simulink model "sistema_fisico_test"  (R2019a)
settings: Solver=VariableStepAuto  StartTime=0.0  StopTime=240  RelTol=1e-3
undefined symbols (not defined in the file): b_cx, b_cy, b_h_eq, b_hb, b_hEb, b_t, b_tb, b_td_eq, b_tw, b_wu, g, H_c, i_h, i_t, K_cy, K_tw, k_wu, l_h0, m_h_eq, M_t, m_td_eq, r_hd, r_td, sigbuilder_block, T_hb_max, T_hEb_max, T_tb_max, x_l0, x_t0, x_td0, y_l0, Y_t0
libraries: simulink x1
settings Model: Creator=Facundo  LastModifiedBy=Facundo

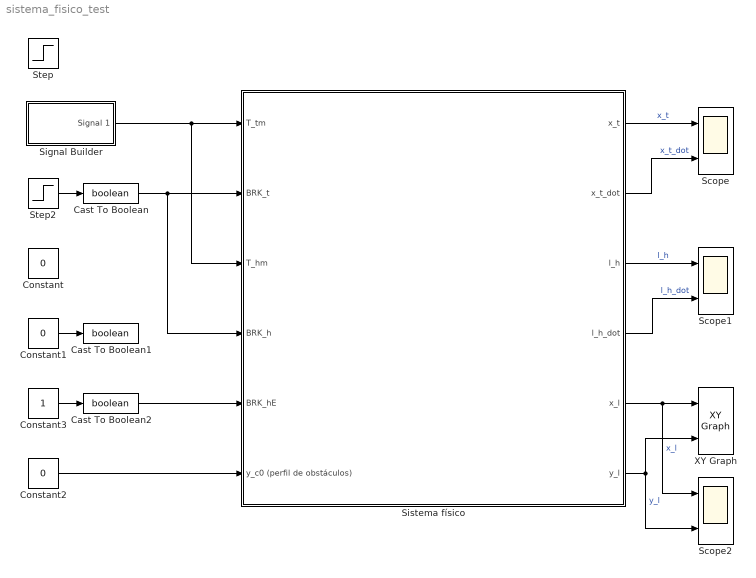
== system sistema_fisico_test ==
  Cast To Boolean : DataTypeConversion  OutDataTypeStr=boolean
  Cast To Boolean1 : DataTypeConversion  OutDataTypeStr=boolean
  Cast To Boolean2 : DataTypeConversion  OutDataTypeStr=boolean
  Constant : Constant  Value=0
  Constant1 : Constant  Value=0  OutDataTypeStr=boolean
  Constant2 : Constant  Value=0
  Constant3 : Constant  OutDataTypeStr=boolean
  Scope : Scope  NumInputPorts=2
  Scope1 : Scope  NumInputPorts=2
  Scope2 : Scope  NumInputPorts=2
  Signal Builder : Subsystem  Tag=STV Subsys  LoadFcn=sigbuilder_block('load');  StartFcn=sigbuilder_block('start');  StopFcn=sigbuilder_block('stop');  ClipboardFcn=sigbuilder_block('clipboard');  mask(Sigbuilder block){tuvar=[0:10]}
      mask help: Simulink:masks:SigbuilderBlock_MD
      mask init:
      | if ~strcmp(get_param(bdroot(gcbh),'SimulationStatus'),'stopped') tuvar = sigbuilder_block('maskInit'); end
      settings: CopyFcn=sigbuilder_block('copy');  DeleteFcn=sigbuilder_block('delete');  ModelCloseFcn=sigbuilder_block('modelClose');  PreSaveFcn=sigbuilder_block('preSave');  PauseFcn=sigbuilder_block('pause');  ContinueFcn=sigbuilder_block('continue');  NameChangeFcn=sigbuilder_block('namechange');  OpenFcn=sigbuilder_block('open',[-1440 -265.714 1440 726.429 ]);  CloseFcn=sigbuilder_block('close');
      mask Display: plot(0, 0, 100, 100,[2, 2, 32, 32, 2], [68, 8, 8, 68, 68],[32, 2], [38, 38], [32, 19, 2],[53, 60, 44], [32, 17, 17, 2],[16, 16, 31, 31]);txt = getActiveGroup(gcbh);text(2, 100, txt,'verticalAlignment', 'top');
  Sistema físico : Subsystem
  Step : Step  Time=0.5  After=1000  SampleTime=0
  Step2 : Step  Time=25  Before=1  After=0  SampleTime=0
  XY Graph : simulink/Sinks/XY Graph  xmin=-100  xmax=100  ymin=-100  ymax=100  st=-1
  wires:
  Constant2/1 -> Sistema físico/6(y_c0 (perfil de obstáculos))
  Constant1/1 -> Cast To Boolean1/1
  Step2/1 -> Cast To Boolean/1
  Sistema físico/2(x_t_dot) -> Scope/2  "x_t_dot"
  Sistema físico/3(l_h) -> Scope1/1  "l_h"
  Sistema físico/5(x_l) -> XY Graph/1, Scope2/1  "x_l"
  Sistema físico/6(y_l) -> Scope2/2, XY Graph/2  "y_l"
  Sistema físico/4(l_h_dot) -> Scope1/2  "l_h_dot"
  Sistema físico/1(x_t) -> Scope/1  "x_t"
  Signal Builder/1(Signal 1) -> Sistema físico/1(T_tm), Sistema físico/3(T_hm)
  Constant3/1 -> Cast To Boolean2/1
  Cast To Boolean2/1 -> Sistema físico/5(BRK_hE)
  Cast To Boolean/1 -> Sistema físico/4(BRK_h), Sistema físico/2(BRK_t)

== system sistema_fisico_test/Signal Builder ==
  Demux : Demux  Tag=STV Demux  Outputs=1
  FromWs : FromWorkspace  Tag=STV FromWs  VariableName=tuvar  SampleTime=0
      SigBuilderData=|
      | common.afterFinalStr = 'Extrapolate'
      | common.sampleTime = 0
      | dataSet.timeRange = [0 60]
      | dataSet.name = 'Group 1'
      | sbobj.Groups.Name = 'Group 1'
      | sbobj.Groups.Signals.Name = 'Signal 1'
      | sbobj.Groups.Signals.XData = [0 1 10 30 60]
      | sbobj.Groups.Signals.YData = [0 1000 1000 0 0]
      | sbobj.Groups.TimeRange = [0 60]
  Signal 1 : Outport  Tag=STV Outport
  wires:
  Demux/1 -> Signal 1/1
  FromWs/1 -> Demux/1

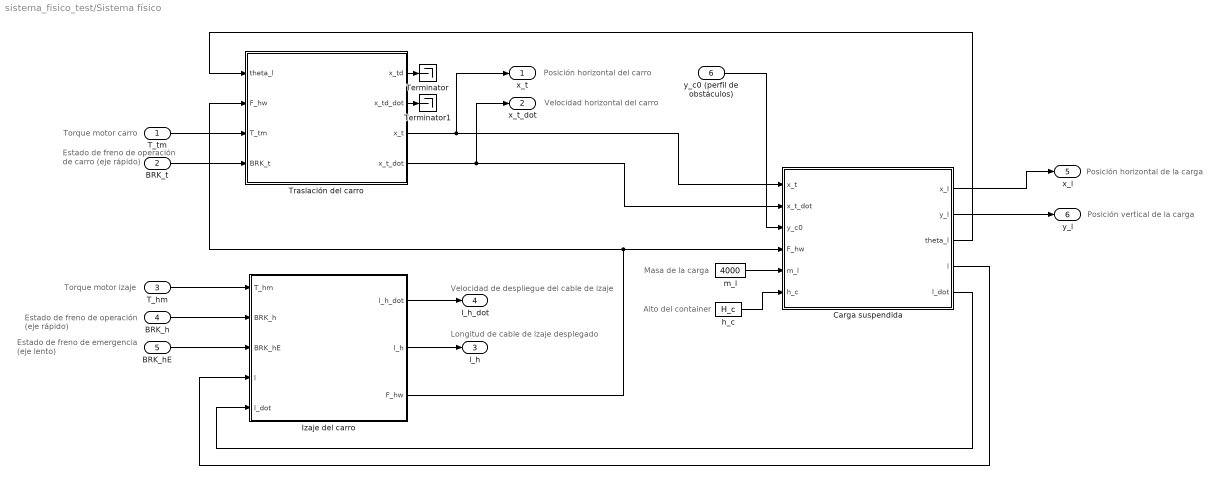
== system sistema_fisico_test/Sistema físico ==
  note: Alto del container
  note: Masa de la carga
  note: Torque motor izaje
  note: Estado de freno de operación
      | (eje rápido)
  note: Estado de freno de emergencia
      | (eje lento)
  note: Estado de freno de
      | operación de carro
      | (eje rápido)
  note: Torque motor carro
  note: Posición vertical de la carga
  note: Posición horizontal de la carga
  note: Longitud de cable de izaje desplegado
  note: Velocidad de despliegue del cable de izaje
  note: Posición horizontal del carro
  note: Velocidad horizontal del carro
  T_tm : Inport
  BRK_t : Inport  Port=2
  T_hm : Inport  Port=3
  BRK_h : Inport  Port=4
  BRK_hE : Inport  Port=5
  y_c0 (perfil de obstáculos) : Inport  Port=6
  Carga suspendida : Subsystem
  Izaje del carro : Subsystem
  Terminator : Terminator
  Terminator1 : Terminator
  Traslación del carro : Subsystem
  h_c : Constant  Value=H_c
  m_l : Constant  Value=4000
  x_t : Outport
  x_t_dot : Outport  Port=2
  l_h : Outport  Port=3
  l_h_dot : Outport  Port=4
  x_l : Outport  Port=5
  y_l : Outport  Port=6
  wires:
  Carga suspendida/5(l_dot) -> Izaje del carro/5(l_dot)
  Traslación del carro/3(x_t) -> x_t/1, Carga suspendida/1(x_t)
  Carga suspendida/2(y_l) -> y_l/1
  Traslación del carro/2(x_td_dot) -> Terminator1/1
  BRK_h/1 -> Izaje del carro/2(BRK_h)
  Izaje del carro/2(l_h) -> l_h/1
  Izaje del carro/1(l_h_dot) -> l_h_dot/1
  m_l/1 -> Carga suspendida/5(m_l)
  Carga suspendida/4(l) -> Izaje del carro/4(l)
  Carga suspendida/1(x_l) -> x_l/1
  Izaje del carro/3(F_hw) -> Traslación del carro/2(F_hw), Carga suspendida/4(F_hw)
  Traslación del carro/4(x_t_dot) -> x_t_dot/1, Carga suspendida/2(x_t_dot)
  BRK_t/1 -> Traslación del carro/4(BRK_t)
  h_c/1 -> Carga suspendida/6(h_c)
  y_c0 (perfil de obstáculos)/1 -> Carga suspendida/3(y_c0)
  BRK_hE/1 -> Izaje del carro/3(BRK_hE)
  Traslación del carro/1(x_td) -> Terminator/1
  T_hm/1 -> Izaje del carro/1(T_hm)
  T_tm/1 -> Traslación del carro/3(T_tm)
  Carga suspendida/3(theta_l) -> Traslación del carro/1(theta_l)

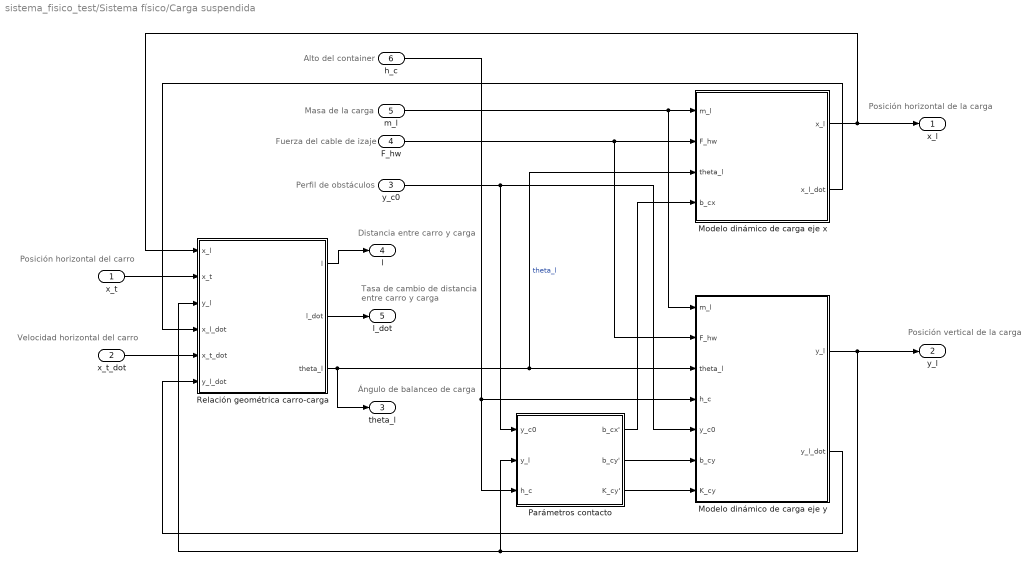
== system sistema_fisico_test/Sistema físico/Carga suspendida ==
  note: Perfil de obstáculos
  note: Posición horizontal del carro
  note: Posición vertical de la carga
  note: Velocidad horizontal del carro
  note: Alto del container
  note: Distancia entre carro y carga
  note: Fuerza del cable de izaje
  note: Ángulo de balanceo de carga
  note: Tasa de cambio de distancia
      | entre carro y carga
  note: Masa de la carga
  note: Posición horizontal de la carga
  x_t : Inport  OutDataTypeStr=double  PortDimensions=1  SampleTime=0
  x_t_dot : Inport  Port=2  OutDataTypeStr=double  PortDimensions=1  SampleTime=0
  y_c0 : Inport  Port=3  OutDataTypeStr=double  PortDimensions=1  SampleTime=0
  F_hw : Inport  Port=4  OutDataTypeStr=double  PortDimensions=1  SampleTime=0
  m_l : Inport  Port=5  OutDataTypeStr=double  PortDimensions=1  SampleTime=0
  h_c : Inport  Port=6  OutDataTypeStr=double  PortDimensions=1  SampleTime=0
  Modelo dinámico de carga eje x : Subsystem
  Modelo dinámico de carga eje y : Subsystem
  Parámetros contacto : Subsystem
  Relación geométrica carro-carga : Subsystem
  x_l : Outport  OutDataTypeStr=double  PortDimensions=1  SampleTime=0
  y_l : Outport  Port=2  OutDataTypeStr=double  PortDimensions=1  SampleTime=0
  theta_l : Outport  Port=3  OutDataTypeStr=double  PortDimensions=1  SampleTime=0
  l : Outport  Port=4  OutDataTypeStr=double  PortDimensions=1  SampleTime=0
  l_dot : Outport  Port=5  OutDataTypeStr=double  PortDimensions=1  SampleTime=0
  wires:
  y_c0/1 -> Parámetros contacto/1(y_c0), Modelo dinámico de carga eje y/5(y_c0)
  m_l/1 -> Modelo dinámico de carga eje y/1(m_l), Modelo dinámico de carga eje x/1(m_l)
  F_hw/1 -> Modelo dinámico de carga eje y/2(F_hw), Modelo dinámico de carga eje x/2(F_hw)
  Relación geométrica carro-carga/2(l_dot) -> l_dot/1
  x_t_dot/1 -> Relación geométrica carro-carga/5(x_t_dot)
  Modelo dinámico de carga eje y/1(y_l) -> y_l/1, Relación geométrica carro-carga/3(y_l), Parámetros contacto/2(y_l)
  h_c/1 -> Modelo dinámico de carga eje y/4(h_c), Parámetros contacto/3(h_c)
  Modelo dinámico de carga eje x/2(x_l_dot) -> Relación geométrica carro-carga/4(x_l_dot)
  Modelo dinámico de carga eje y/2(y_l_dot) -> Relación geométrica carro-carga/6(y_l_dot)
  x_t/1 -> Relación geométrica carro-carga/2(x_t)
  Modelo dinámico de carga eje x/1(x_l) -> x_l/1, Relación geométrica carro-carga/1(x_l)
  Relación geométrica carro-carga/3(theta_l) -> theta_l/1, Modelo dinámico de carga eje x/3(theta_l), Modelo dinámico de carga eje y/3(theta_l)  "theta_l"
  Parámetros contacto/1(b_cx') -> Modelo dinámico de carga eje x/4(b_cx)
  Parámetros contacto/2(b_cy') -> Modelo dinámico de carga eje y/6(b_cy)
  Parámetros contacto/3(K_cy') -> Modelo dinámico de carga eje y/7(K_cy)
  Relación geométrica carro-carga/1(l) -> l/1

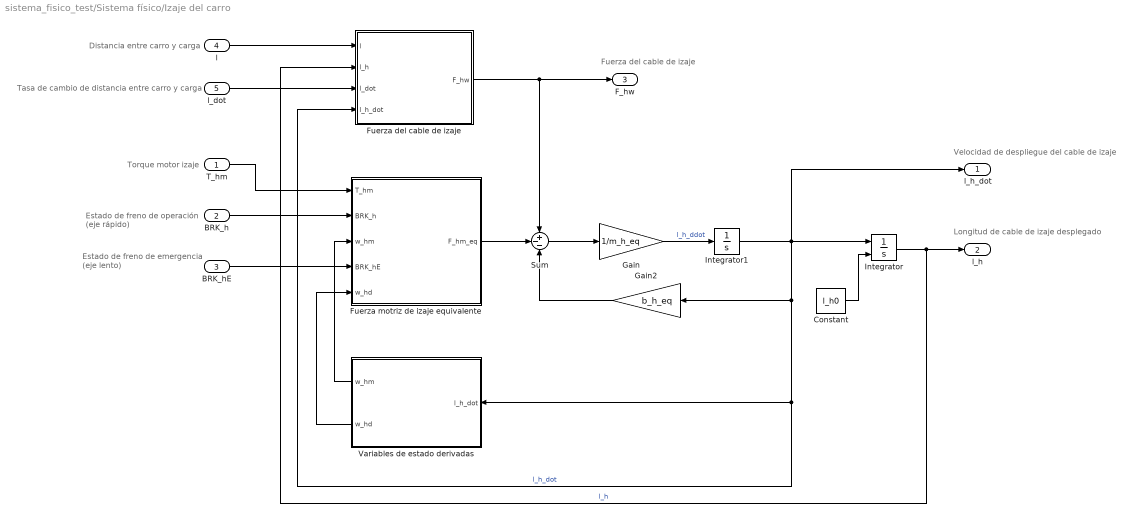
== system sistema_fisico_test/Sistema físico/Izaje del carro ==
  note: Longitud de cable de izaje desplegado
  note: Velocidad de despliegue del cable de izaje
  note: Torque motor izaje
  note: Estado de freno de emergencia
      | (eje lento)
  note: Tasa de cambio de distancia entre carro y carga
  note: Estado de freno de operación
      | (eje rápido)
  note: Distancia entre carro y carga
  note: Fuerza del cable de izaje
  T_hm : Inport
  BRK_h : Inport  Port=2
  BRK_hE : Inport  Port=3
  l : Inport  Port=4
  l_dot : Inport  Port=5
  Constant : Constant  Value=l_h0
  Fuerza del cable de izaje : Subsystem
  Fuerza motriz de izaje equivalente : Subsystem
  Gain : Gain  Gain=1/m_h_eq
  Gain2 : Gain  Gain=b_h_eq
  Integrator : Integrator  InitialConditionSource=external
  Integrator1 : Integrator
  Sum : Sum  Inputs=+--
  Variables de estado derivadas : Subsystem
  l_h_dot : Outport
  l_h : Outport  Port=2
  F_hw : Outport  Port=3
  wires:
  Integrator/1 -> l_h/1, Fuerza del cable de izaje/2(l_h)  "l_h"
  Integrator1/1 -> l_h_dot/1, Fuerza del cable de izaje/4(l_h_dot), Variables de estado derivadas/1(l_h_dot), Gain2/1, Integrator/1  "l_h_dot"
  T_hm/1 -> Fuerza motriz de izaje equivalente/1(T_hm)
  l/1 -> Fuerza del cable de izaje/1(l)
  l_dot/1 -> Fuerza del cable de izaje/3(l_dot)
  Fuerza del cable de izaje/1(F_hw) -> F_hw/1, Sum/1
  Gain2/1 -> Sum/3
  Fuerza motriz de izaje equivalente/1(F_hm_eq) -> Sum/2
  Variables de estado derivadas/1(w_hm) -> Fuerza motriz de izaje equivalente/3(w_hm)
  Sum/1 -> Gain/1
  Variables de estado derivadas/2(w_hd) -> Fuerza motriz de izaje equivalente/5(w_hd)
  BRK_h/1 -> Fuerza motriz de izaje equivalente/2(BRK_h)
  BRK_hE/1 -> Fuerza motriz de izaje equivalente/4(BRK_hE)
  Gain/1 -> Integrator1/1  "l_h_ddot"
  Constant/1 -> Integrator/2

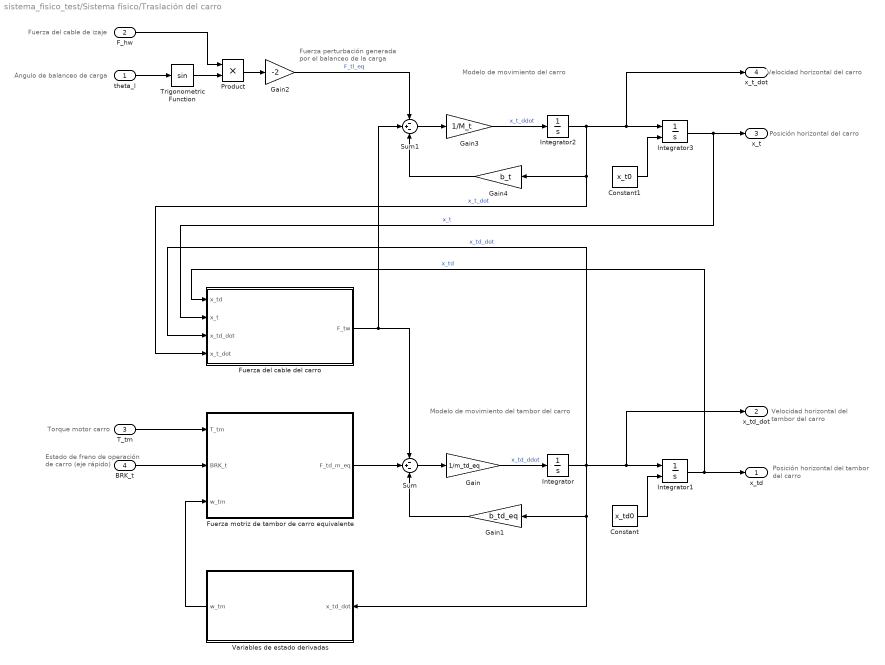
== system sistema_fisico_test/Sistema físico/Traslación del carro ==
  note: Velocidad horizontal
      | del tambor del carro
  note: Modelo de movimiento del tambor del carro
  note: Modelo de movimiento del carro
  note: Velocidad horizontal del carro
  note: Estado de freno de
      | operación de carro
      | (eje rápido)
  note: Fuerza del cable de izaje
  note: Fuerza perturbación generada
      | por el balanceo de la carga
  note: Posición horizontal del carro
  note: Torque motor carro
  note: Ángulo de balanceo de carga
  note: Posición horizontal
      | del tambor del carro
  theta_l : Inport  OutDataTypeStr=double  PortDimensions=1  SampleTime=0
  F_hw : Inport  Port=2  OutDataTypeStr=double  PortDimensions=1  SampleTime=0
  T_tm : Inport  Port=3
  BRK_t : Inport  Port=4
  Constant : Constant  Value=x_td0
  Constant1 : Constant  Value=x_t0
  Fuerza del cable del carro : Subsystem
  Fuerza motriz de tambor de carro equivalente : Subsystem
  Gain : Gain  Gain=1/m_td_eq
  Gain1 : Gain  Gain=b_td_eq
  Gain2 : Gain  Gain=-2
  Gain3 : Gain  Gain=1/M_t
  Gain4 : Gain  Gain=b_t
  Integrator : Integrator
  Integrator1 : Integrator  InitialConditionSource=external
  Integrator2 : Integrator
  Integrator3 : Integrator  InitialConditionSource=external
  Product : Product
  Sum : Sum  Inputs=-+-
  Sum1 : Sum  Inputs=-+-
  Trigonometric Function : Trigonometry
  Variables de estado derivadas : Subsystem
  x_td : Outport  OutDataTypeStr=double  PortDimensions=1  SampleTime=0
  x_td_dot : Outport  Port=2  OutDataTypeStr=double  PortDimensions=1  SampleTime=0
  x_t : Outport  Port=3  OutDataTypeStr=double  PortDimensions=1  SampleTime=0
  x_t_dot : Outport  Port=4  OutDataTypeStr=double  PortDimensions=1  SampleTime=0
  wires:
  Integrator1/1 -> x_td/1, Fuerza del cable del carro/1(x_td)  "x_td"
  Gain3/1 -> Integrator2/1  "x_t_ddot"
  Fuerza del cable del carro/1(F_tw) -> Sum1/2, Sum/1
  Sum/1 -> Gain/1
  Integrator/1 -> Fuerza del cable del carro/3(x_td_dot), Variables de estado derivadas/1(x_td_dot), Gain1/1, x_td_dot/1, Integrator1/1  "x_td_dot"
  F_hw/1 -> Product/1
  Fuerza motriz de tambor de carro equivalente/1(F_td_m_eq) -> Sum/2
  Constant/1 -> Integrator1/2
  Gain1/1 -> Sum/3
  Integrator2/1 -> Fuerza del cable del carro/4(x_t_dot), Gain4/1, x_t_dot/1, Integrator3/1  "x_t_dot"
  Sum1/1 -> Gain3/1
  theta_l/1 -> Trigonometric Function/1
  Gain4/1 -> Sum1/3
  Integrator3/1 -> x_t/1, Fuerza del cable del carro/2(x_t)  "x_t"
  Gain2/1 -> Sum1/1  "F_tl_eq"
  T_tm/1 -> Fuerza motriz de tambor de carro equivalente/1(T_tm)
  BRK_t/1 -> Fuerza motriz de tambor de carro equivalente/2(BRK_t)
  Variables de estado derivadas/1(w_tm) -> Fuerza motriz de tambor de carro equivalente/3(w_tm)
  Constant1/1 -> Integrator3/2
  Trigonometric Function/1 -> Product/2
  Product/1 -> Gain2/1
  Gain/1 -> Integrator/1  "x_td_ddot"

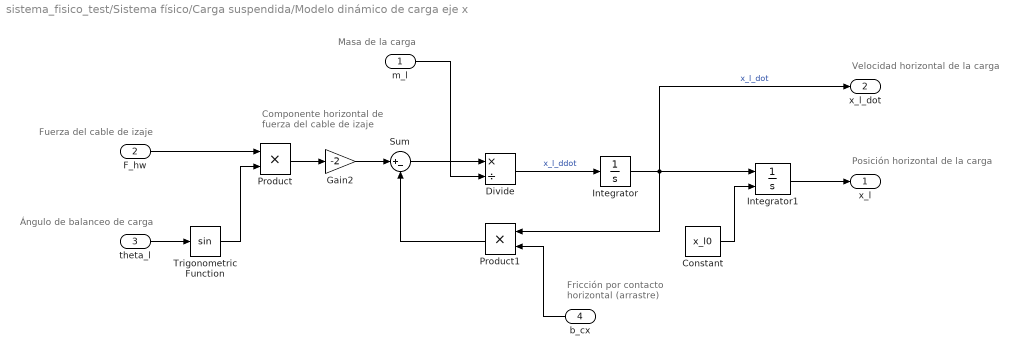
== system sistema_fisico_test/Sistema físico/Carga suspendida/Modelo dinámico de carga eje x ==
  note: Componente horizontal de
      | fuerza del cable de izaje
  note: Posición horizontal de la carga
  note: Velocidad horizontal de la carga
  note: Fuerza del cable de izaje
  note: Masa de la carga
  note: Fricción por contacto
      | horizontal (arrastre)
  note: Ángulo de balanceo de carga
  m_l : Inport  OutDataTypeStr=double  PortDimensions=1  SampleTime=0
  F_hw : Inport  Port=2  OutDataTypeStr=double  PortDimensions=1  SampleTime=0
  theta_l : Inport  Port=3  OutDataTypeStr=double  PortDimensions=1  SampleTime=0
  b_cx : Inport  Port=4  OutDataTypeStr=double  PortDimensions=1  SampleTime=0
  Constant : Constant  Value=x_l0
  Divide : Product  Inputs=*/
  Gain2 : Gain  Gain=-2
  Integrator : Integrator
  Integrator1 : Integrator  InitialConditionSource=external
  Product : Product
  Product1 : Product
  Sum : Sum  Inputs=|+-
  Trigonometric Function : Trigonometry
  x_l : Outport  OutDataTypeStr=double  PortDimensions=1  SampleTime=0
  x_l_dot : Outport  Port=2  OutDataTypeStr=double  PortDimensions=1  SampleTime=0
  wires:
  F_hw/1 -> Product/1
  Product1/1 -> Sum/2
  theta_l/1 -> Trigonometric Function/1
  b_cx/1 -> Product1/2
  Sum/1 -> Divide/1
  Integrator/1 -> x_l_dot/1, Integrator1/1, Product1/1  "x_l_dot"
  Product/1 -> Gain2/1
  Divide/1 -> Integrator/1  "x_l_ddot"
  Constant/1 -> Integrator1/2
  Integrator1/1 -> x_l/1
  Gain2/1 -> Sum/1
  m_l/1 -> Divide/2
  Trigonometric Function/1 -> Product/2

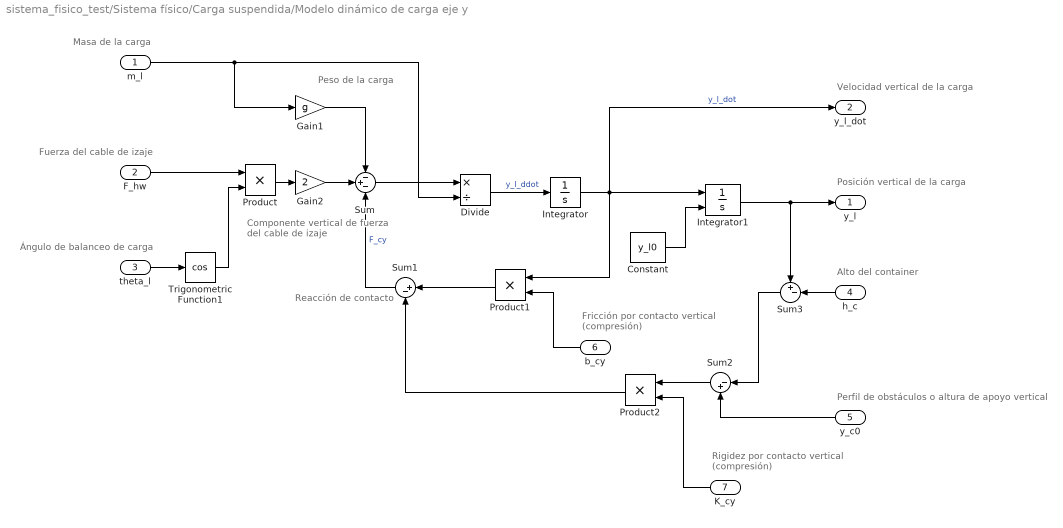
== system sistema_fisico_test/Sistema físico/Carga suspendida/Modelo dinámico de carga eje y ==
  note: Reacción de contacto
  note: Peso de la carga
  note: Componente vertical de
      | fuerza del cable de izaje
  note: Posición vertical de la carga
  note: Velocidad vertical de la carga
  note: Fricción por contacto
      | vertical (compresión)
  note: Rigidez por contacto
      | vertical (compresión)
  note: Masa de la carga
  note: Fuerza del cable de izaje
  note: Perfil de obstáculos o altura de apoyo vertical
  note: Alto del container
  note: Ángulo de balanceo de carga
  m_l : Inport  OutDataTypeStr=double  PortDimensions=1  SampleTime=0
  F_hw : Inport  Port=2  OutDataTypeStr=double  PortDimensions=1  SampleTime=0
  theta_l : Inport  Port=3  OutDataTypeStr=double  PortDimensions=1  SampleTime=0
  h_c : Inport  Port=4  OutDataTypeStr=double  PortDimensions=1  SampleTime=0
  y_c0 : Inport  Port=5  OutDataTypeStr=double  PortDimensions=1  SampleTime=0
  b_cy : Inport  Port=6  OutDataTypeStr=double  PortDimensions=1  SampleTime=0
  K_cy : Inport  Port=7  OutDataTypeStr=double  PortDimensions=1  SampleTime=0
  Constant : Constant  Value=y_l0
  Divide : Product  Inputs=*/
  Gain1 : Gain  Gain=g
  Gain2 : Gain  Gain=2
  Integrator : Integrator
  Integrator1 : Integrator  InitialConditionSource=external
  Product : Product
  Product1 : Product
  Product2 : Product
  Sum : Sum  Inputs=-+-
  Sum1 : Sum  Inputs=|+-
  Sum2 : Sum  Inputs=|-+
  Sum3 : Sum  Inputs=+-|
  Trigonometric Function1 : Trigonometry  Operator=cos
  y_l : Outport  OutDataTypeStr=double  PortDimensions=1  SampleTime=0
  y_l_dot : Outport  Port=2  OutDataTypeStr=double  PortDimensions=1  SampleTime=0
  wires:
  F_hw/1 -> Product/1
  theta_l/1 -> Trigonometric Function1/1
  b_cy/1 -> Product1/2
  Integrator/1 -> y_l_dot/1, Integrator1/1, Product1/1  "y_l_dot"
  Divide/1 -> Integrator/1  "y_l_ddot"
  Constant/1 -> Integrator1/2
  Integrator1/1 -> y_l/1, Sum3/1
  Product/1 -> Gain2/1
  Product1/1 -> Sum1/1
  Sum1/1 -> Sum/3  "F_cy"
  Gain1/1 -> Sum/1
  y_c0/1 -> Sum2/2
  Sum2/1 -> Product2/1
  K_cy/1 -> Product2/2
  Product2/1 -> Sum1/2
  Gain2/1 -> Sum/2
  Sum/1 -> Divide/1
  m_l/1 -> Gain1/1, Divide/2
  h_c/1 -> Sum3/2
  Sum3/1 -> Sum2/1
  Trigonometric Function1/1 -> Product/2

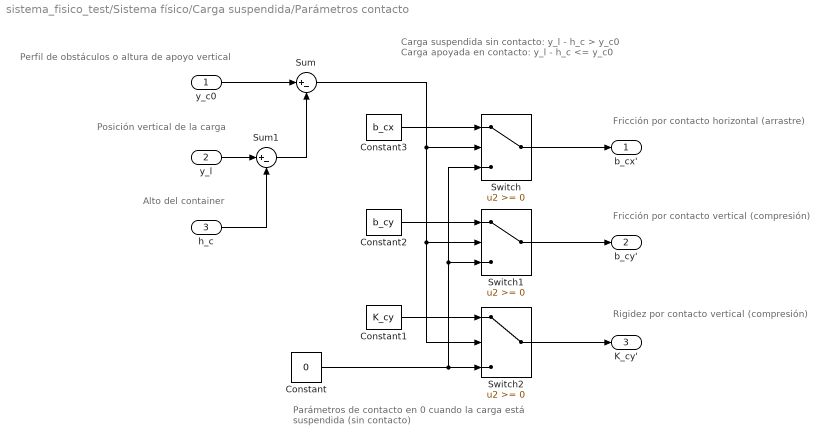
== system sistema_fisico_test/Sistema físico/Carga suspendida/Parámetros contacto ==
  note: Fricción por contacto horizontal (arrastre)
  note: Fricción por contacto vertical (compresión)
  note: Rigidez por contacto vertical (compresión)
  note: Perfil de obstáculos o altura de apoyo vertical
  note: Posición vertical de la carga
  note: Alto del container
  note: Parámetros de contacto en 0
      | cuando la carga está suspendida (sin contacto)
  note: Carga suspendida sin contacto: y_l - h_c > y_c0
      | Carga apoyada en contacto: y_l - h_c <= y_c0
  y_c0 : Inport  OutDataTypeStr=double  PortDimensions=1  SampleTime=0
  y_l : Inport  Port=2  OutDataTypeStr=double  PortDimensions=1  SampleTime=0
  h_c : Inport  Port=3  OutDataTypeStr=double  PortDimensions=1  SampleTime=0
  Constant : Constant  Value=0
  Constant1 : Constant  Value=K_cy
  Constant2 : Constant  Value=b_cy
  Constant3 : Constant  Value=b_cx
  Sum : Sum  Inputs=|+-
  Sum1 : Sum  Inputs=|+-
  Switch : Switch
  Switch1 : Switch
  Switch2 : Switch
  b_cx' : Outport  OutDataTypeStr=double  PortDimensions=1  SampleTime=0
  b_cy' : Outport  Port=2  OutDataTypeStr=double  PortDimensions=1  SampleTime=0
  K_cy' : Outport  Port=3  OutDataTypeStr=double  PortDimensions=1  SampleTime=0
  wires:
  y_c0/1 -> Sum/1
  Constant2/1 -> Switch1/1
  Constant1/1 -> Switch2/1
  Switch/1 -> b_cx'/1
  Sum/1 -> Switch1/2, Switch2/2, Switch/2
  Switch2/1 -> K_cy'/1
  Switch1/1 -> b_cy'/1
  Constant/1 -> Switch/3, Switch1/3, Switch2/3
  Constant3/1 -> Switch/1
  Sum1/1 -> Sum/2
  y_l/1 -> Sum1/1
  h_c/1 -> Sum1/2

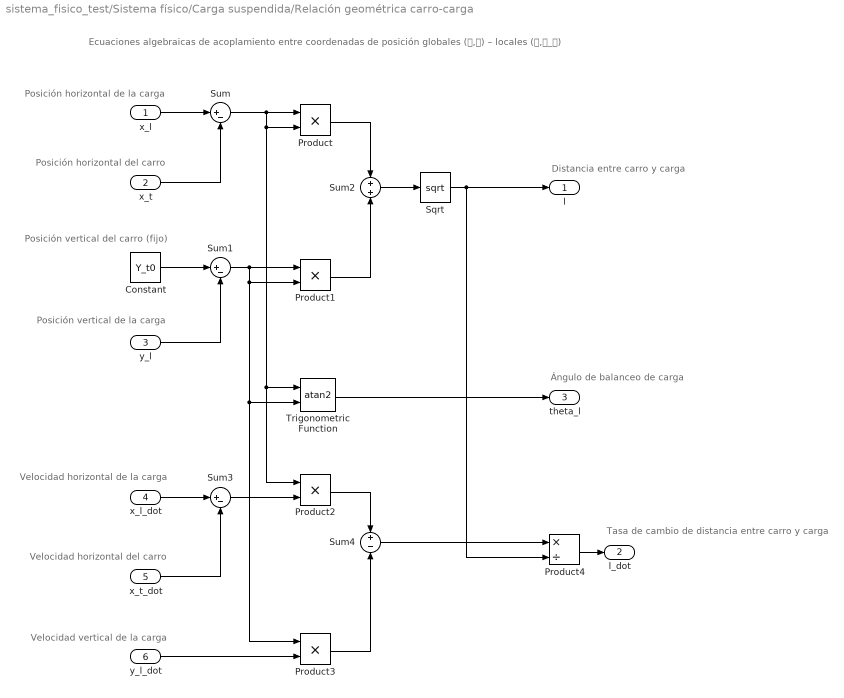
== system sistema_fisico_test/Sistema físico/Carga suspendida/Relación geométrica carro-carga ==
  note: Ecuaciones algebraicas de acoplamiento entre coordenadas de posición globales (𝑥,𝑦) – locales (𝑙,𝜃_𝑙)
  note: Posición horizontal de la carga
  note: Posición horizontal del carro
  note: Posición vertical del carro (fijo)
  note: Posición vertical de la carga
  note: Distancia entre carro y carga
  note: Tasa de cambio de distancia entre carro y carga
  note: Ángulo de balanceo de carga
  note: Velocidad horizontal de la carga
  note: Velocidad horizontal del carro
  note: Velocidad vertical de la carga
  x_l : Inport
  x_t : Inport  Port=2
  y_l : Inport  Port=3
  x_l_dot : Inport  Port=4
  x_t_dot : Inport  Port=5
  y_l_dot : Inport  Port=6
  Constant : Constant  Value=Y_t0
  Product{,1..3} (4 alike) : Product
  Product4 : Product  Inputs=*/
  Sqrt : Sqrt  SaturateOnIntegerOverflow=on
  Sum : Sum  Inputs=|+-
  Sum1 : Sum  Inputs=|+-
  Sum2 : Sum  Inputs=+|+
  Sum3 : Sum  Inputs=|+-
  Sum4 : Sum  Inputs=+|-
  Trigonometric Function : Trigonometry  Operator=atan2
  l : Outport
  l_dot : Outport  Port=2
  theta_l : Outport  Port=3
  wires:
  x_t/1 -> Sum/2
  x_l/1 -> Sum/1
  Sum/1 -> Product/1, Product2/1, Trigonometric Function/1, Product/2
  Product/1 -> Sum2/1
  y_l/1 -> Sum1/2
  Sum1/1 -> Product1/1, Product3/1, Trigonometric Function/2, Product1/2
  Constant/1 -> Sum1/1
  Product1/1 -> Sum2/2
  Sum2/1 -> Sqrt/1
  Trigonometric Function/1 -> theta_l/1
  x_l_dot/1 -> Sum3/1
  x_t_dot/1 -> Sum3/2
  Sum3/1 -> Product2/2
  y_l_dot/1 -> Product3/2
  Product2/1 -> Sum4/1
  Product3/1 -> Sum4/2
  Sum4/1 -> Product4/1
  Product4/1 -> l_dot/1
  Sqrt/1 -> Product4/2, l/1

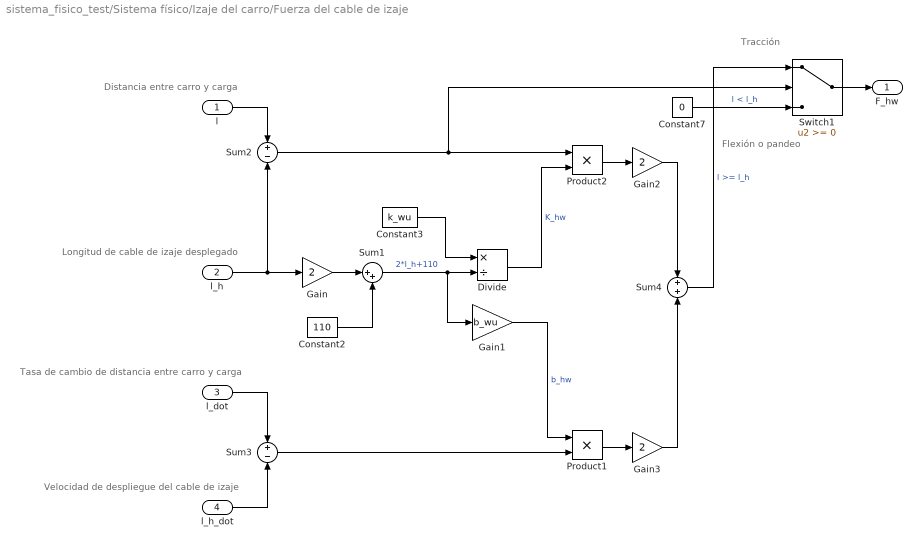
== system sistema_fisico_test/Sistema físico/Izaje del carro/Fuerza del cable de izaje ==
  note: Flexión o pandeo
  note: Tracción
  note: Distancia entre carro y carga
  note: Tasa de cambio de distancia entre carro y carga
  note: Longitud de cable de izaje desplegado
  note: Velocidad de despliegue del cable de izaje
  l : Inport
  l_h : Inport  Port=2
  l_dot : Inport  Port=3
  l_h_dot : Inport  Port=4
  Constant2 : Constant  Value=110
  Constant3 : Constant  Value=k_wu
  Constant7 : Constant  Value=0
  Divide : Product  Inputs=*/
  Gain : Gain  Gain=2
  Gain1 : Gain  Gain=b_wu
  Gain2 : Gain  Gain=2
  Gain3 : Gain  Gain=2
  Product1 : Product
  Product2 : Product
  Sum1 : Sum  Inputs=|++
  Sum2 : Sum  Inputs=+-
  Sum3 : Sum  Inputs=+-
  Sum4 : Sum
  Switch1 : Switch
  F_hw : Outport
  wires:
  l_dot/1 -> Sum3/1
  Constant2/1 -> Sum1/2
  Sum1/1 -> Gain1/1, Divide/2  "2*l_h+110"
  l/1 -> Sum2/1
  Product1/1 -> Gain3/1
  Sum3/1 -> Product1/2
  l_h_dot/1 -> Sum3/2
  l_h/1 -> Gain/1, Sum2/2
  Divide/1 -> Product2/2  "K_hw"
  Sum2/1 -> Switch1/2, Product2/1
  Constant3/1 -> Divide/1
  Gain1/1 -> Product1/1  "b_hw"
  Product2/1 -> Gain2/1
  Switch1/1 -> F_hw/1
  Sum4/1 -> Switch1/1  "l >= l_h"
  Constant7/1 -> Switch1/3  "l < l_h"
  Gain/1 -> Sum1/1
  Gain2/1 -> Sum4/1
  Gain3/1 -> Sum4/2

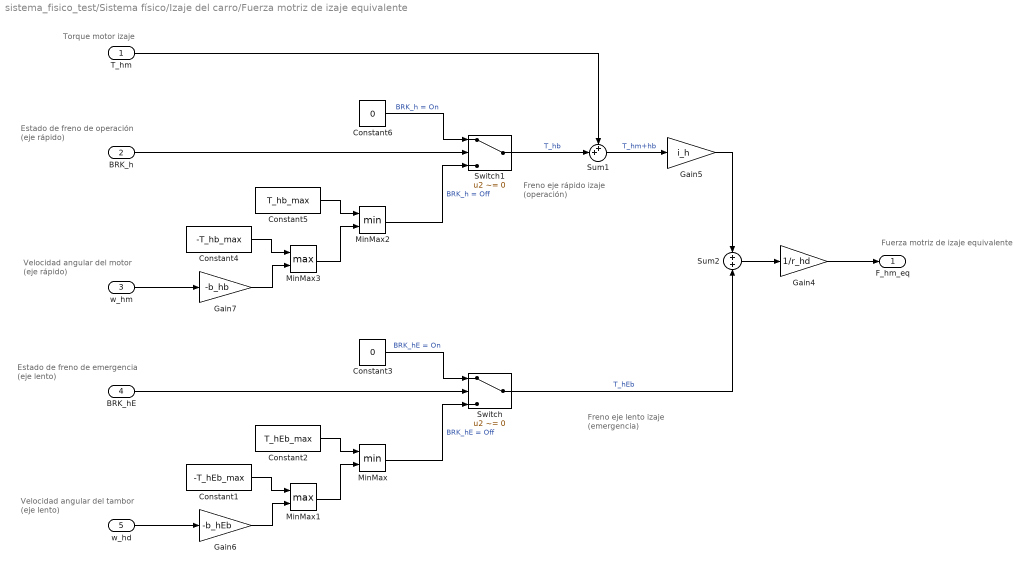
== system sistema_fisico_test/Sistema físico/Izaje del carro/Fuerza motriz de izaje equivalente ==
  note: Fuerza motriz de izaje equivalente
  note: Torque motor izaje
  note: Freno eje lento izaje
      | (emergencia)
  note: Freno eje rápido izaje
      | (operación)
  note: Estado de freno de operación
      | (eje rápido)
  note: Estado de freno de emergencia
      | (eje lento)
  note: Velocidad angular del tambor
      | (eje lento)
  note: Velocidad angular del motor
      | (eje rápido)
  T_hm : Inport
  BRK_h : Inport  Port=2  OutDataTypeStr=boolean
  w_hm : Inport  Port=3
  BRK_hE : Inport  Port=4  OutDataTypeStr=boolean
  w_hd : Inport  Port=5
  Constant1 : Constant  Value=-T_hEb_max
  Constant2 : Constant  Value=T_hEb_max
  Constant3 : Constant  Value=0
  Constant4 : Constant  Value=-T_hb_max
  Constant5 : Constant  Value=T_hb_max
  Constant6 : Constant  Value=0
  Gain4 : Gain  Gain=1/r_hd
  Gain5 : Gain  Gain=i_h
  Gain6 : Gain  Gain=-b_hEb
  Gain7 : Gain  Gain=-b_hb
  MinMax : MinMax  Inputs=2
  MinMax1 : MinMax  Function=max  Inputs=2
  MinMax2 : MinMax  Inputs=2
  MinMax3 : MinMax  Function=max  Inputs=2
  Sum1 : Sum  Inputs=++|
  Sum2 : Sum  Inputs=2
  Switch : Switch  Criteria=u2 ~= 0
  Switch1 : Switch  Criteria=u2 ~= 0
  F_hm_eq : Outport
  wires:
  MinMax3/1 -> MinMax2/2
  MinMax1/1 -> MinMax/2
  Constant1/1 -> MinMax1/1
  MinMax2/1 -> Switch1/3  "BRK_h = Off"
  Gain5/1 -> Sum2/1
  Constant4/1 -> MinMax3/1
  T_hm/1 -> Sum1/1
  w_hm/1 -> Gain7/1
  Constant5/1 -> MinMax2/1
  w_hd/1 -> Gain6/1
  Gain7/1 -> MinMax3/2
  BRK_h/1 -> Switch1/2
  Constant6/1 -> Switch1/1  "BRK_h = On"
  MinMax/1 -> Switch/3  "BRK_hE = Off"
  Sum1/1 -> Gain5/1  "T_hm+hb"
  Switch1/1 -> Sum1/2  "T_hb"
  Constant3/1 -> Switch/1  "BRK_hE = On"
  BRK_hE/1 -> Switch/2
  Constant2/1 -> MinMax/1
  Gain6/1 -> MinMax1/2
  Gain4/1 -> F_hm_eq/1
  Sum2/1 -> Gain4/1
  Switch/1 -> Sum2/2  "T_hEb"

== system sistema_fisico_test/Sistema físico/Izaje del carro/Variables de estado derivadas ==
  note: Velocidad angular del tambor
  note: Caja reductora
      | entre motor y tambor
  note: Velocidad angular del motor
  note: Velocidad de despliegue del cable de izaje
  l_h_dot : Inport
  Gain1 : Gain  Gain=-2/r_hd
  Gain3 : Gain  Gain=i_h
  w_hm : Outport
  w_hd : Outport  Port=2
  wires:
  Gain1/1 -> w_hd/1, Gain3/1  "w_hd"
  l_h_dot/1 -> Gain1/1
  Gain3/1 -> w_hm/1  "w_hm"

== system sistema_fisico_test/Sistema físico/Traslación del carro/Fuerza del cable del carro ==
  note: Posición de tambor del carro
  note: Velocidad del tambor del carro
  note: Posición del carro
  note: Velocidad del carro
  note: Fuerza del cable del carro
  x_td : Inport
  x_t : Inport  Port=2
  x_td_dot : Inport  Port=3
  x_t_dot : Inport  Port=4
  Gain : Gain  Gain=K_tw
  Gain1 : Gain  Gain=b_tw
  Sum2 : Sum  Inputs=+-
  Sum3 : Sum  Inputs=+-
  Sum4 : Sum
  F_tw : Outport
  wires:
  x_td_dot/1 -> Sum3/1
  x_td/1 -> Sum2/1
  x_t_dot/1 -> Sum3/2
  x_t/1 -> Sum2/2
  Sum4/1 -> F_tw/1
  Gain/1 -> Sum4/1
  Sum2/1 -> Gain/1
  Gain1/1 -> Sum4/2
  Sum3/1 -> Gain1/1

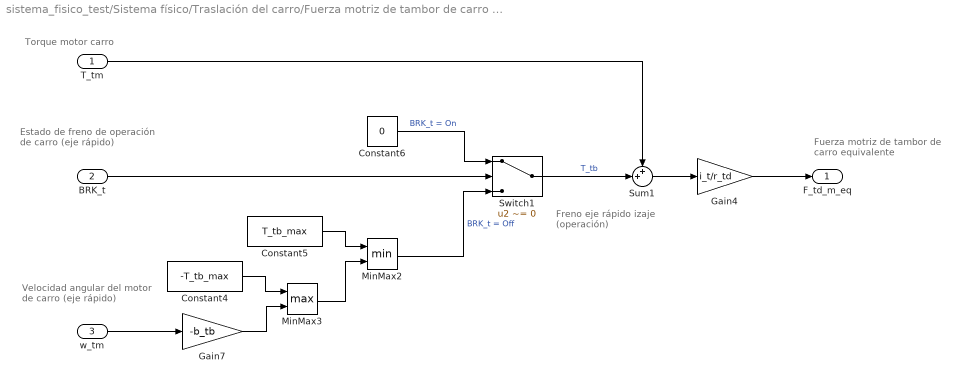
== system sistema_fisico_test/Sistema físico/Traslación del carro/Fuerza motriz de tambor de carro equivalente ==
  note: Fuerza motriz de tambor
      | de carro equivalente
  note: Torque motor carro
  note: Freno eje rápido izaje
      | (operación)
  note: Estado de freno de
      | operación de carro
      | (eje rápido)
  note: Velocidad angular
      | del motor de carro
      | (eje rápido)
  T_tm : Inport
  BRK_t : Inport  Port=2  OutDataTypeStr=boolean
  w_tm : Inport  Port=3
  Constant4 : Constant  Value=-T_tb_max
  Constant5 : Constant  Value=T_tb_max
  Constant6 : Constant  Value=0
  Gain4 : Gain  Gain=i_t/r_td
  Gain7 : Gain  Gain=-b_tb
  MinMax2 : MinMax  Inputs=2
  MinMax3 : MinMax  Function=max  Inputs=2
  Sum1 : Sum  Inputs=++|
  Switch1 : Switch  Criteria=u2 ~= 0
  F_td_m_eq : Outport
  wires:
  MinMax3/1 -> MinMax2/2
  MinMax2/1 -> Switch1/3  "BRK_t = Off"
  Constant4/1 -> MinMax3/1
  T_tm/1 -> Sum1/1
  w_tm/1 -> Gain7/1
  Constant5/1 -> MinMax2/1
  Gain7/1 -> MinMax3/2
  BRK_t/1 -> Switch1/2
  Constant6/1 -> Switch1/1  "BRK_t = On"
  Sum1/1 -> Gain4/1
  Switch1/1 -> Sum1/2  "T_tb"
  Gain4/1 -> F_td_m_eq/1

== system sistema_fisico_test/Sistema físico/Traslación del carro/Variables de estado derivadas ==
  note: Radio del tambor
  note: Caja reductora
      | entre motor y tambor
  note: Velocidad angular del motor del carro
  note: Velocidad de la carga sin balanceo
  x_td_dot : Inport
  Gain1 : Gain  Gain=1/r_td
  Gain3 : Gain  Gain=i_t
  w_tm : Outport
  wires:
  Gain1/1 -> Gain3/1  "w_td"
  x_td_dot/1 -> Gain1/1
  Gain3/1 -> w_tm/1  "w_tm"
